simulink model "mdl2"  (Simulink 5.0)
settings: Solver=ode1  StartTime=0.0  StopTime=5  FixedStep=0.01  RelTol=1e-3
values from neighbouring files (symbols this model uses):
  amp = 5    [data.mat]
  eps1 = 1    [data.mat]
  eps2 = 0.5    [data.mat]
libraries: simulink x1
settings Model: LastModifiedBy=student  ExtModeMexFile=rti_comm  ExtModeArmWhenConnect=off  BlockReductionOpt=off  ConditionallyExecuteInputs=off  OptimizeBlockIOStorage=off  RTWSystemTargetFile=rti1102.tlc  RTWTemplateMakefile=rti1102.tmf  RTWMakeCommand=make_rti  RTWRetainRTWFile=on

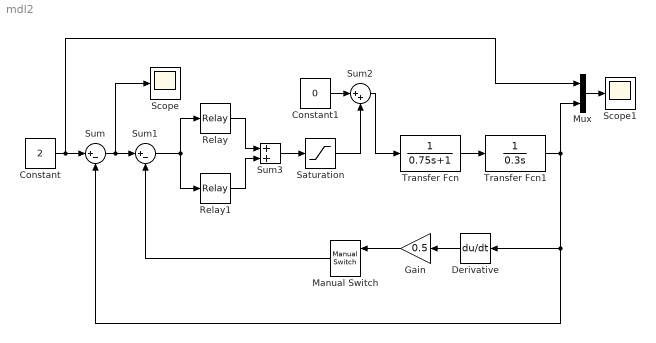
== system mdl2 ==
  Constant : Constant  Value=2
  Constant1 : Constant  Value=0
  Derivative : Derivative  Orientation=left
  Gain : Gain  Orientation=left  Gain=0.5  SaturateOnIntegerOverflow=on
  Manual Switch : simulink/Signal Routing/Manual Switch  Orientation=left  sw=0  action=0
  Mux : Mux  Inputs=2
  Relay : Relay  OnSwitchValue=eps1  OffSwitchValue=eps2  OnOutputValue=amp
  Relay1 : Relay  OnSwitchValue=-eps2  OffSwitchValue=-eps1  OnOutputValue=0  OffOutputValue=-amp
  Saturation : Saturate  UpperLimit=5  LowerLimit=-5
  Scope : Scope
  Scope1 : Scope
  Sum : Sum  Inputs=|+-  SaturateOnIntegerOverflow=on
  Sum1 : Sum  Inputs=|+-  SaturateOnIntegerOverflow=on
  Sum2 : Sum  Inputs=|++  SaturateOnIntegerOverflow=on
  Sum3 : Sum  SaturateOnIntegerOverflow=on
  Transfer Fcn : TransferFcn  Denominator=[0.75 1]
  Transfer Fcn1 : TransferFcn  Denominator=[0.3 0]
  wires:
  Constant/1 -> Sum/1, Mux/1
  Sum/1 -> Sum1/1, Scope/1
  Sum1/1 -> Relay/1, Relay1/1
  Saturation/1 -> Sum2/2
  Constant1/1 -> Sum2/1
  Transfer Fcn/1 -> Transfer Fcn1/1
  Sum2/1 -> Transfer Fcn/1
  Transfer Fcn1/1 -> Mux/2, Derivative/1, Sum/2
  Derivative/1 -> Gain/1
  Gain/1 -> Manual Switch/1
  Manual Switch/1 -> Sum1/2
  Mux/1 -> Scope1/1
  Sum3/1 -> Saturation/1
  Relay1/1 -> Sum3/2
  Relay/1 -> Sum3/1
